simulink model "test"  (R2018b)
settings: Solver=VariableStepAuto  StartTime=0.0  StopTime=simTime  RelTol=1e-3
values from neighbouring files (symbols this model uses):
  dt = 2    [testSimBayes_ts.m]
  iniPt = ((xMax-xMin).*rand(2,1) + xMin)    [testSimBayes_ts.m]
  simTime = 15    [testSimBayes_ts.m]
libraries: bayesianAscent_cl x1
settings Model: Creator=asiddiq2  LastModifiedBy=asiddiq2

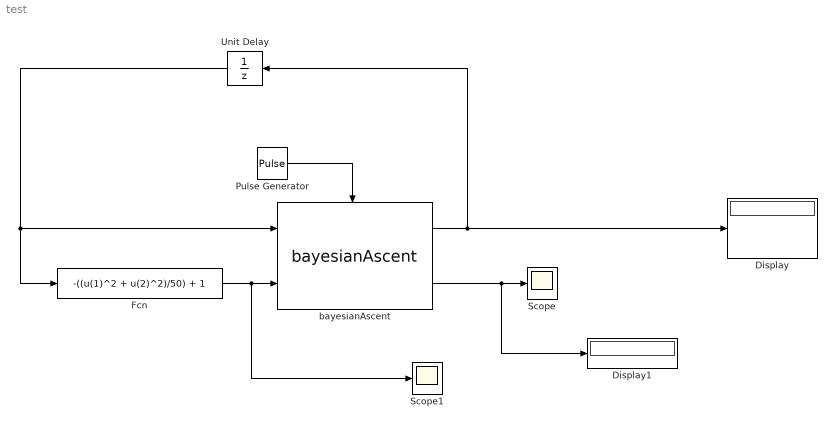
== system test ==
  Display : Display
  Display1 : Display
  Fcn : Fcn  Expr=-((u(1)^2 + u(2)^2)/50) + 1
  Pulse Generator : DiscretePulseGenerator  PulseType=Time based  Period=dt  PulseWidth=5
  Scope : Scope
  Scope1 : Scope
  Unit Delay : UnitDelay  InitialCondition=iniPt  SampleTime=-1
  bayesianAscent : bayesianAscent_cl/bayesianAscent  gpTrain=trainDsgns  gpTrainFval=trainFval  iniOptHyp=trainOpHyp  noiseVars=noiseVar  desLims=designLimits  gamma=gamma  beta=beta  iniTauPerc=iniTauPerc  maxIter=ceil(simTime/dt)
  wires:
  bayesianAscent/1 -> Display/1, Unit Delay/1
  Pulse Generator/1 -> bayesianAscent/Enable
  Fcn/1 -> Scope1/1, bayesianAscent/2
  bayesianAscent/2 -> Display1/1, Scope/1
  Unit Delay/1 -> Fcn/1, bayesianAscent/1
